simulink model "fixedEEControlR2016a"  (Simulink 8.8)
settings: Solver=ode5  StartTime=0.0  StopTime=inf  FixedStep=0.01  RelTol=1e-3  EnableMultiTasking=on
InitFcn:
  | initFixedEEControl
values from neighbouring files (symbols this model uses):
  WBTConfigRobot = WBToolbox.Configuration    [initEndEffectorControl.m]    (also in initFixedEEControl.m)
undefined symbols (not defined in the file or in its folder): CONFIG, GAINS
libraries: WBToolboxLibrary x19
settings Model: SuppressorTable=22 serialization::archive 11 0 3 0 0 0 11 0  Creator=yeshi  LastModifiedBy=icub  NumberOfSteps=50
settings DataIOCC: LimitDataPoints=off  SaveFormat=Dataset  SignalLoggingSaveFormat=Dataset
settings DebuggingCC: UnderspecifiedInitializationDetection=Simplified  MergeDetectMultiDrivingBlocksExec=error  FcnCallInpInsideContextMsg=error  StateNameClashWarn=none
settings HardwareCC: ProdBitPerPointer=64  ProdBitPerSizeT=64  ProdBitPerPtrDiffT=64  ProdLargestAtomicFloat=Float  ProdIntDivRoundTo=Zero  ProdEndianess=LittleEndian  ProdWordSize=64  ProdHWDeviceType=Intel->x86-64 (Windows64)
settings ModelReferenceCC: PropagateSignalLabelsOutOfModel=on
settings GRTTargetCC: CombineOutputUpdateFcns=on  GRTInterface=off

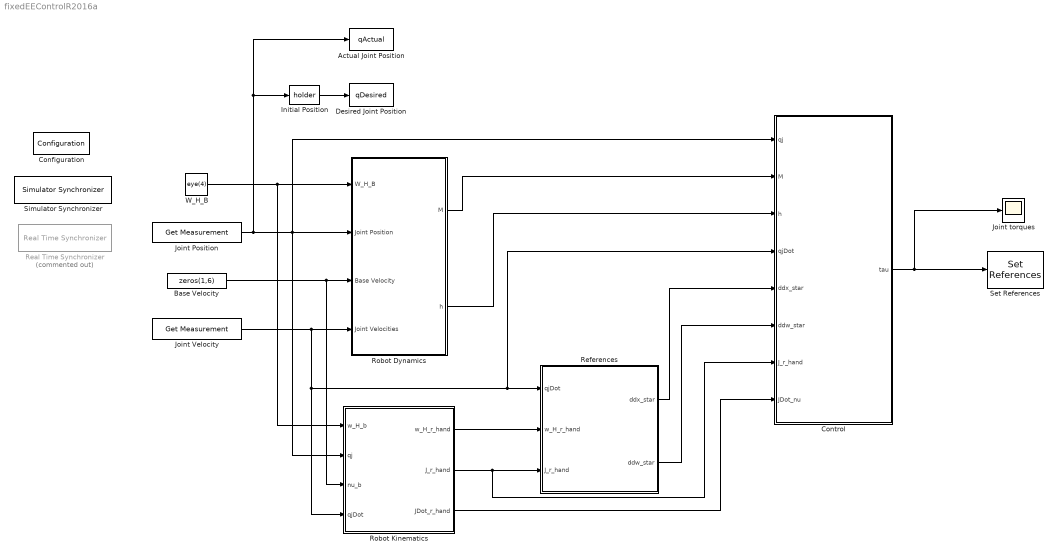
== system fixedEEControlR2016a ==
  Actual Joint Position : ToWorkspace  VariableName=qActual  SaveFormat=Timeseries  SampleTime=-1
  "Base Velocity " : Constant  Value=zeros(1,6)
  Configuration : WBToolboxLibrary/Utilities/Configuration  ConfigSource=Workspace  ConfigObject='WBTConfigRobot'  RobotName='icub'  UrdfFile='model.urdf'  ControlledJoints={'l_elbow','l_shoulder_pitch','torso_roll'}  ControlBoardsNames={'left_arm','right_arm','torso'}  LocalName='WBT'  GravityVector=[0,0,-9.81]
  Control : Subsystem
  Desired Joint Position : ToWorkspace  VariableName=qDesired  SaveFormat=Timeseries  SampleTime=-1
  "Initial Position " : WBToolboxLibrary/Utilities/holder 
  Joint Position : WBToolboxLibrary/wholeBodyStates/Get Measurement  measuredType=Joints Position
  Joint Velocity : WBToolboxLibrary/wholeBodyStates/Get Measurement  measuredType=Joints Velocity
  Joint torques : Scope
  Real Time Synchronizer : WBToolboxLibrary/Utilities/Real Time Synchronizer  Commented=on  period=0.01
  References : Subsystem
  Robot Dynamics : Subsystem
  Robot Kinematics : Subsystem
  Set References : WBToolboxLibrary/wholeBodyActuators/Set References  controlType=Torque  refSpeed=50
  Simulator Synchronizer : WBToolboxLibrary/Utilities/Simulator Synchronizer  period=0.01  serverPortName='/clock/rpc'  clientPortName='/WBT_synchronizer/rpc:o'
  "W_H_B " : Constant  Value=eye(4)
  wires:
  Joint Position/1 -> Robot Kinematics/2(qj), Control/1(qj), Robot Dynamics/2(Joint Position), Actual Joint Position/1, "Initial Position "/1
  Joint Velocity/1 -> Robot Kinematics/4(qjDot), Control/4(qjDot), References/1(qjDot), Robot Dynamics/4(" Joint Velocities ")
  "W_H_B "/1 -> Robot Kinematics/1(w_H_b), Robot Dynamics/1(W_H_B)
  "Base Velocity "/1 -> Robot Kinematics/3(nu_b), Robot Dynamics/3(Base Velocity)
  Robot Kinematics/1(w_H_r_hand) -> References/2(w_H_r_hand)
  Control/1(tau) -> Set References/1, Joint torques/1
  Robot Kinematics/3(JDot_r_hand) -> Control/8(JDot_nu)
  Robot Kinematics/2(J_r_hand) -> References/3(J_r_hand), Control/7(J_r_hand)
  References/1(ddx_star) -> Control/5(ddx_star)
  Robot Dynamics/2(h) -> Control/3(h)
  References/2(ddw_star) -> Control/6(ddw_star)
  "Initial Position "/1 -> Desired Joint Position/1
  Robot Dynamics/1(M) -> Control/2(M)

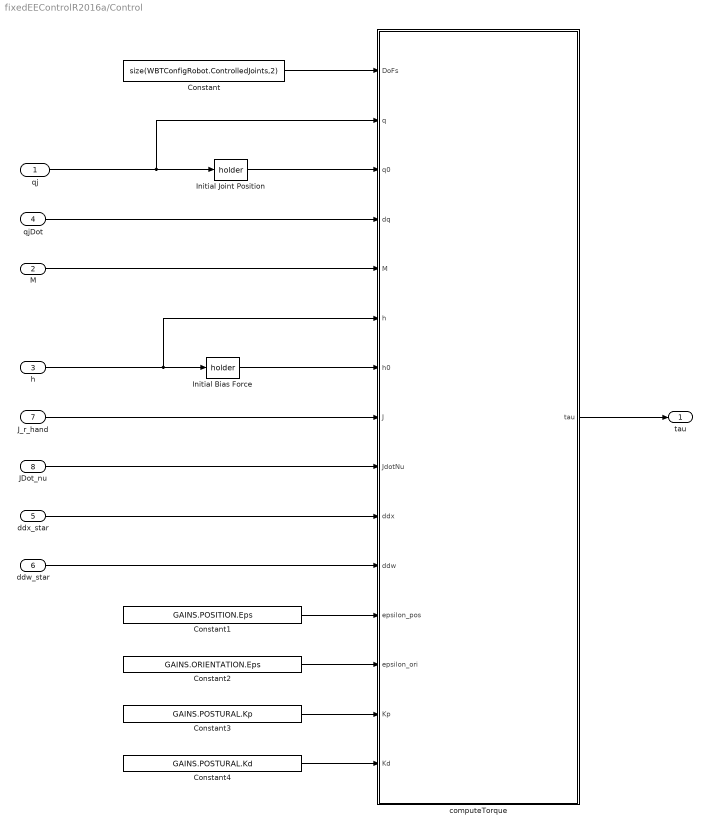
== system fixedEEControlR2016a/Control ==
  qj : Inport
  M : Inport  Port=2
  h : Inport  Port=3
  qjDot : Inport  Port=4
  ddx_star : Inport  Port=5
  ddw_star : Inport  Port=6
  J_r_hand : Inport  Port=7
  JDot_nu : Inport  Port=8
  Constant : Constant  Value=size(WBTConfigRobot.ControlledJoints,2)
  Constant1 : Constant  Value=GAINS.POSITION.Eps
  Constant2 : Constant  Value=GAINS.ORIENTATION.Eps
  Constant3 : Constant  Value=GAINS.POSTURAL.Kp
  Constant4 : Constant  Value=GAINS.POSTURAL.Kd
  Initial Bias Force : WBToolboxLibrary/Utilities/holder 
  Initial Joint Position : WBToolboxLibrary/Utilities/holder 
  computeTorque : MATLAB Function  TreatAsAtomicUnit=on
  tau : Outport
  wires:
  ddx_star/1 -> computeTorque/10(ddx)
  qj/1 -> Initial Joint Position/1, computeTorque/2(q)
  qjDot/1 -> computeTorque/4(dq)
  JDot_nu/1 -> computeTorque/9(JdotNu)
  Constant/1 -> computeTorque/1(DoFs)
  computeTorque/1(tau) -> tau/1
  h/1 -> computeTorque/6(h), Initial Bias Force/1
  Initial Bias Force/1 -> computeTorque/7(h0)
  Initial Joint Position/1 -> computeTorque/3(q0)
  J_r_hand/1 -> computeTorque/8(J)
  M/1 -> computeTorque/5(M)
  ddw_star/1 -> computeTorque/11(ddw)
  Constant1/1 -> computeTorque/12(epsilon_pos)
  Constant2/1 -> computeTorque/13(epsilon_ori)
  Constant3/1 -> computeTorque/14(Kp)
  Constant4/1 -> computeTorque/15(Kd)

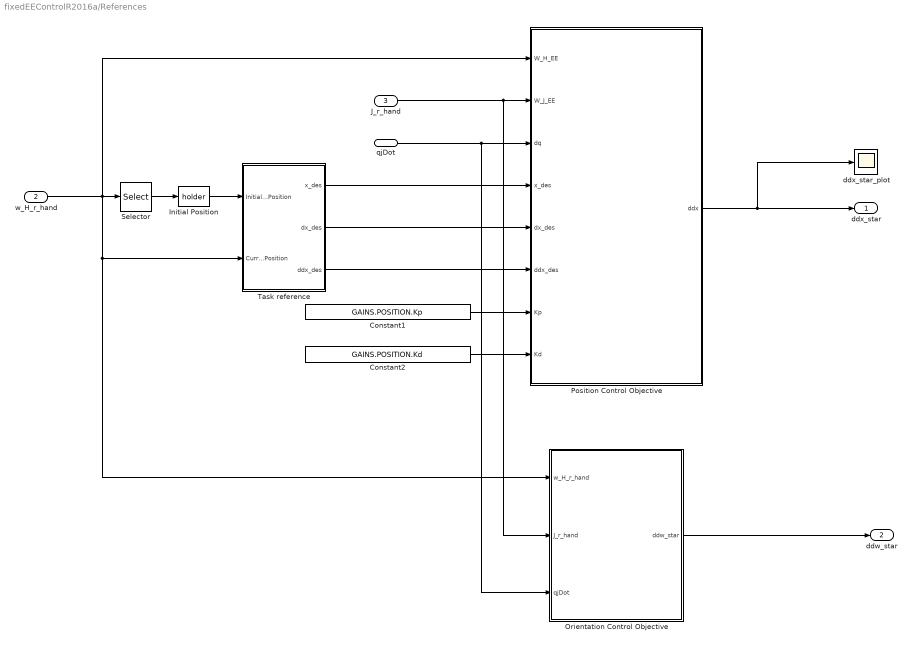
== system fixedEEControlR2016a/References ==
  qjDot : Inport
  w_H_r_hand : Inport  Port=2
  J_r_hand : Inport  Port=3
  Constant1 : Constant  Value=GAINS.POSITION.Kp
  Constant2 : Constant  Value=GAINS.POSITION.Kd
  "Initial Position " : WBToolboxLibrary/Utilities/holder 
  Orientation Control Objective : Subsystem
  Position Control Objective : MATLAB Function  TreatAsAtomicUnit=on
  Selector : Selector  NumberOfDimensions=2  InputPortWidth=3  IndexOptions=Index vector (dialog),Index vector (dialog)  Indices=[1 2 3],4  OutputSizes=1,1
  Task reference : Subsystem
  ddx_star_plot : Scope
  ddx_star : Outport
  ddw_star : Outport  Port=2
  wires:
  J_r_hand/1 -> Orientation Control Objective/2(J_r_hand), Position Control Objective/2(W_J_EE)
  Task reference/1(x_des) -> Position Control Objective/4(x_des)
  Task reference/2(dx_des) -> Position Control Objective/5(dx_des)
  Task reference/3(ddx_des) -> Position Control Objective/6(ddx_des)
  "Initial Position "/1 -> Task reference/1(Initial Position)
  Position Control Objective/1(ddx) -> ddx_star/1, ddx_star_plot/1
  Selector/1 -> "Initial Position "/1
  qjDot/1 -> Orientation Control Objective/3(qjDot), Position Control Objective/3(dq)
  w_H_r_hand/1 -> Selector/1, Position Control Objective/1(W_H_EE), Orientation Control Objective/1(w_H_r_hand), Task reference/2(Current Position)
  Constant1/1 -> Position Control Objective/7(Kp)
  Constant2/1 -> Position Control Objective/8(Kd)
  Orientation Control Objective/1(ddw_star) -> ddw_star/1

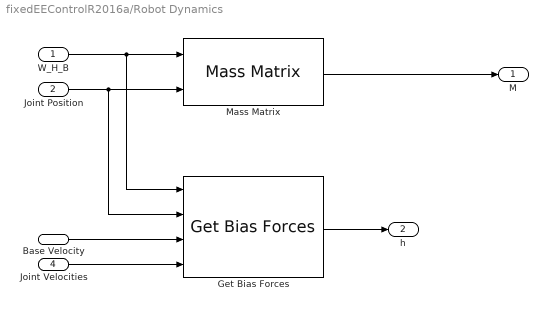
== system fixedEEControlR2016a/Robot Dynamics ==
  W_H_B : Inport
  Joint Position : Inport  Port=2
  Base Velocity : Inport  Port=3
  " Joint Velocities " : Inport  Port=4
  Get Bias Forces : WBToolboxLibrary/wholeBodyModel/Dynamics/Get Bias Forces
  Mass Matrix : WBToolboxLibrary/wholeBodyModel/Dynamics/Mass Matrix
  M : Outport
  h : Outport  Port=2
  wires:
  Joint Position/1 -> Mass Matrix/2, Get Bias Forces/2
  " Joint Velocities "/1 -> Get Bias Forces/4
  Get Bias Forces/1 -> h/1
  W_H_B/1 -> Mass Matrix/1, Get Bias Forces/1
  Base Velocity/1 -> Get Bias Forces/3
  Mass Matrix/1 -> M/1

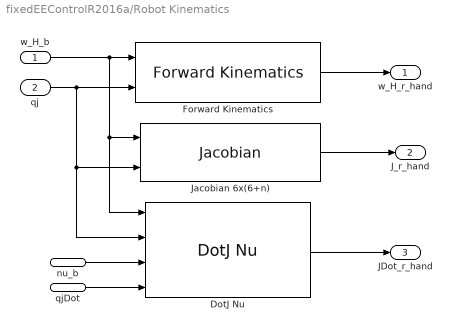
== system fixedEEControlR2016a/Robot Kinematics ==
  w_H_b : Inport
  qj : Inport  Port=2
  nu_b : Inport  Port=3
  qjDot : Inport  Port=4
  DotJ Nu : WBToolboxLibrary/wholeBodyModel/Jacobians/DotJ Nu  frameName=CONFIG.EE
  Forward Kinematics : WBToolboxLibrary/wholeBodyModel/Kinematics/Forward Kinematics  frameName=CONFIG.EE
  Jacobian 6x(6+n) : WBToolboxLibrary/wholeBodyModel/Jacobians/Jacobian  frameName=CONFIG.EE
  w_H_r_hand : Outport
  J_r_hand : Outport  Port=2
  JDot_r_hand : Outport  Port=3
  wires:
  w_H_b/1 -> DotJ Nu/1, Jacobian 6x(6+n)/1, Forward Kinematics/1
  qj/1 -> DotJ Nu/2, Jacobian 6x(6+n)/2, Forward Kinematics/2
  qjDot/1 -> DotJ Nu/4
  nu_b/1 -> DotJ Nu/3
  Jacobian 6x(6+n)/1 -> J_r_hand/1
  Forward Kinematics/1 -> w_H_r_hand/1
  DotJ Nu/1 -> JDot_r_hand/1

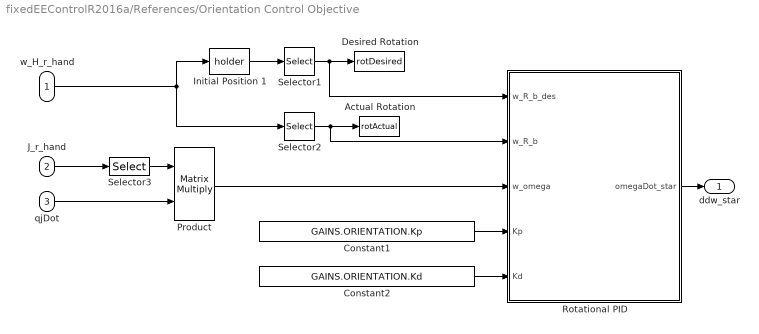
== system fixedEEControlR2016a/References/Orientation Control Objective ==
  w_H_r_hand : Inport
  J_r_hand : Inport  Port=2
  qjDot : Inport  Port=3
  Actual Rotation : ToWorkspace  VariableName=rotActual  SaveFormat=Timeseries  SampleTime=-1
  Constant1 : Constant  Value=GAINS.ORIENTATION.Kp
  Constant2 : Constant  Value=GAINS.ORIENTATION.Kd
  Desired Rotation : ToWorkspace  VariableName=rotDesired  SaveFormat=Timeseries  SampleTime=-1
  Initial Position 1 : WBToolboxLibrary/Utilities/holder 
  Product : Product  Multiplication=Matrix(*)
  Rotational PID : MATLAB Function  TreatAsAtomicUnit=on
  Selector1 : Selector  NumberOfDimensions=2  InputPortWidth=4  IndexOptions=Index vector (dialog),Index vector (dialog)  Indices=[1:3],[1:3]  OutputSizes=1,1
  Selector2 : Selector  NumberOfDimensions=2  InputPortWidth=4  IndexOptions=Index vector (dialog),Index vector (dialog)  Indices=[1:3],[1:3]  OutputSizes=1,1
  Selector3 : Selector  NumberOfDimensions=2  InputPortWidth=4  IndexOptions=Index vector (dialog),Index vector (dialog)  Indices=[4:6],[7:6+13]  OutputSizes=1,1
  ddw_star : Outport
  wires:
  Selector2/1 -> Rotational PID/2(w_R_b), Actual Rotation/1
  Rotational PID/1(omegaDot_star) -> ddw_star/1
  Selector1/1 -> Desired Rotation/1, Rotational PID/1(w_R_b_des)
  w_H_r_hand/1 -> Selector2/1, Initial Position 1/1
  Initial Position 1/1 -> Selector1/1
  Constant1/1 -> Rotational PID/4(Kp)
  Constant2/1 -> Rotational PID/5(Kd)
  J_r_hand/1 -> Selector3/1
  Selector3/1 -> Product/1
  qjDot/1 -> Product/2
  Product/1 -> Rotational PID/3(w_omega)

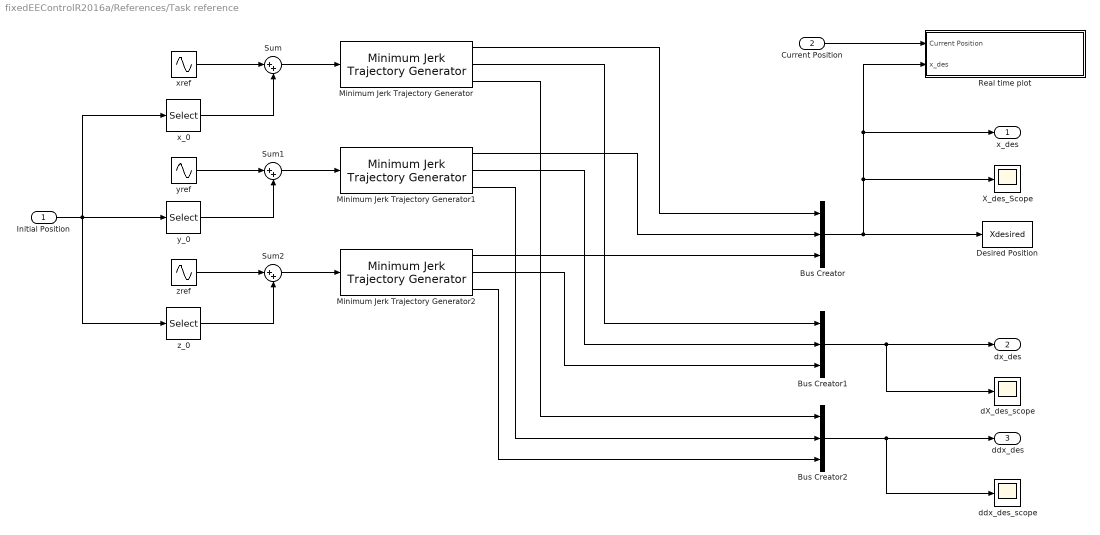
== system fixedEEControlR2016a/References/Task reference ==
  Initial Position : Inport
  Current Position : Inport  Port=2
  Bus Creator : BusCreator  Inputs=3
  Bus Creator1 : BusCreator  Inputs=3
  Bus Creator2 : BusCreator  Inputs=3
  Desired Position : ToWorkspace  VariableName=Xdesired  SaveFormat=Timeseries  SampleTime=-1
  Minimum Jerk Trajectory Generator : WBToolboxLibrary/Utilities/Minimum Jerk Trajectory Generator  externalSettlingTime=off  settlingTime=3  sampleTime=0.01  resetOnSettlingTime=off  firstDerivatives=on  secondDerivatives=on  explicitInitialValue=off
  Minimum Jerk Trajectory Generator1 : WBToolboxLibrary/Utilities/Minimum Jerk Trajectory Generator  externalSettlingTime=off  settlingTime=3  sampleTime=0.01  resetOnSettlingTime=off  firstDerivatives=on  secondDerivatives=on  explicitInitialValue=off
  Minimum Jerk Trajectory Generator2 : WBToolboxLibrary/Utilities/Minimum Jerk Trajectory Generator  externalSettlingTime=off  settlingTime=3  sampleTime=0.01  resetOnSettlingTime=off  firstDerivatives=on  secondDerivatives=on  explicitInitialValue=off
  Real time plot : Subsystem
  Sum : Sum  Inputs=|++
  Sum1 : Sum  Inputs=|++
  Sum2 : Sum  Inputs=|++
  X_des_Scope : Scope
  dX_des_scope : Scope
  ddx_des_scope : Scope
  x_0 : Selector  InputPortWidth=3  IndexOptions=Index vector (dialog)  Indices=[1]  OutputSizes=1
  xref : Sin  Amplitude=0  SampleTime=0
  y_0 : Selector  InputPortWidth=3  IndexOptions=Index vector (dialog)  Indices=[2]  OutputSizes=1
  yref : Sin  Amplitude=0.075  SampleTime=0
  z_0 : Selector  InputPortWidth=3  IndexOptions=Index vector (dialog)  Indices=[3]  OutputSizes=1
  zref : Sin  Amplitude=0.075  Phase=pi/2  SampleTime=0
  x_des : Outport
  dx_des : Outport  Port=2
  ddx_des : Outport  Port=3
  wires:
  Minimum Jerk Trajectory Generator2/2 -> Bus Creator1/3
  Sum2/1 -> Minimum Jerk Trajectory Generator2/1
  Minimum Jerk Trajectory Generator2/1 -> Bus Creator/3
  Minimum Jerk Trajectory Generator/3 -> Bus Creator2/1
  yref/1 -> Sum1/1
  Minimum Jerk Trajectory Generator/1 -> Bus Creator/1
  Minimum Jerk Trajectory Generator1/3 -> Bus Creator2/2
  y_0/1 -> Sum1/2
  Sum1/1 -> Minimum Jerk Trajectory Generator1/1
  Minimum Jerk Trajectory Generator2/3 -> Bus Creator2/3
  Bus Creator1/1 -> dx_des/1, dX_des_scope/1
  zref/1 -> Sum2/1
  Minimum Jerk Trajectory Generator1/2 -> Bus Creator1/2
  Bus Creator2/1 -> ddx_des/1, ddx_des_scope/1
  Bus Creator/1 -> Desired Position/1, Real time plot/2(x_des), x_des/1, X_des_Scope/1
  Minimum Jerk Trajectory Generator1/1 -> Bus Creator/2
  xref/1 -> Sum/1
  Minimum Jerk Trajectory Generator/2 -> Bus Creator1/1
  Sum/1 -> Minimum Jerk Trajectory Generator/1
  z_0/1 -> Sum2/2
  Initial Position/1 -> x_0/1, y_0/1, z_0/1
  x_0/1 -> Sum/2
  Current Position/1 -> Real time plot/1(Current Position)

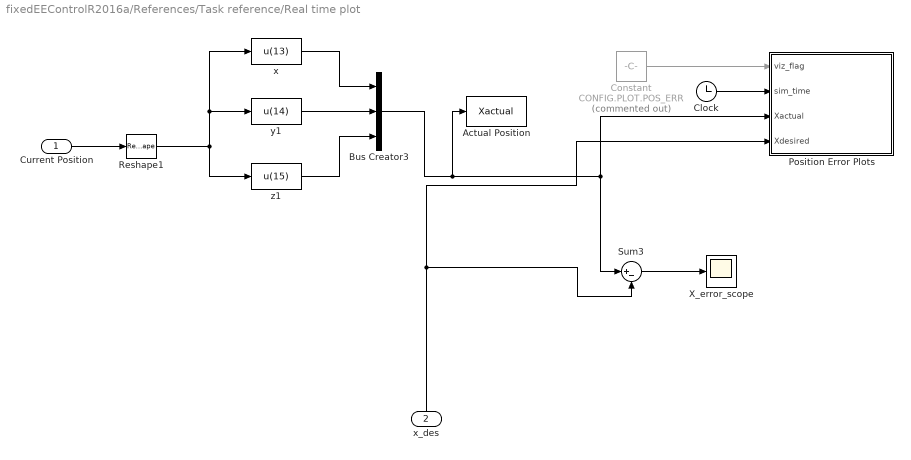
== system fixedEEControlR2016a/References/Task reference/Real time plot ==
  Current Position : Inport
  x_des : Inport  Port=2
  Actual Position : ToWorkspace  VariableName=Xactual  SaveFormat=Timeseries  SampleTime=-1
  Bus Creator3 : BusCreator  Inputs=3
  Clock : Clock
  Constant : Constant  Commented=on  Value=CONFIG.PLOT.POS_ERR
  "Position Error Plots " : MATLAB Function  TreatAsAtomicUnit=on
  Reshape1 : Reshape
  Sum3 : Sum  Inputs=|+-
  X_error_scope : Scope
  x : Fcn  Expr=u(13)
  y1 : Fcn  Expr=u(14)
  z1 : Fcn  Expr=u(15)
  wires:
  x_des/1 -> Sum3/2, "Position Error Plots "/4(Xdesired)
  Current Position/1 -> Reshape1/1
  Reshape1/1 -> x/1, y1/1, z1/1
  x/1 -> Bus Creator3/1
  y1/1 -> Bus Creator3/2
  z1/1 -> Bus Creator3/3
  Clock/1 -> "Position Error Plots "/2(sim_time)
  Bus Creator3/1 -> Actual Position/1, Sum3/1, "Position Error Plots "/3(Xactual)
  Constant/1 -> "Position Error Plots "/1(viz_flag)
  Sum3/1 -> X_error_scope/1

== matlab function References/Position Control Objective ==
  data: W_H_EE input double; ddx output double; W_J_EE input double; dq input double; x_des input double; dx_des input double; ddx_des input double; Kp input double; Kd input double
function ddx = controlObjective(W_H_EE,W_J_EE,dq,x_des,dx_des,ddx_des,Kp,Kd)
   
    x  = W_H_EE(1:3,4)-x_des;
    dx = W_J_EE(1:3,7:end)*dq-dx_des;
    
    ddx = ddx_des-Kp*x-Kd*dx; 

end

== matlab function Control/computeTorque ==
  data: DoFs input double; q input double; q0 input double; dq input double; M input double; h input double; h0 input double; J input double; JdotNu input double; ddx input double; tau output double; ddw input double; epsilon_pos input double; epsilon_ori input double; Kp input double; Kd input double
function tau   = computeTorque(DoFs,q,q0,dq,M,h,h0,J,JdotNu,ddx,ddw,epsilon_pos,epsilon_ori,Kp,Kd)

    Dofs = 13;
    
    Sb = zeros(Dofs,6);
    Ss = eye(Dofs);
    S = [Sb Ss]';

    ddX = [ddx' ddw']';

    %%Position Task
    lambda_pos = (J(1:3,:)/M)*S;
    alpha_pos = pinvDamped(lambda_pos,epsilon_pos);
    
    tau_pos = alpha_pos*(ddX(1:3) - JdotNu(1:3) + (J(1:3,:)/M)*h);
    
    nullspace_pos = eye(size(lambda_pos,2)) - alpha_pos*lambda_pos;
    
    %%Orientation Task
    lambda_ori = (J(4:6,:)/M)*S*nullspace_pos;
    alpha_ori = pinvDamped(lambda_ori,epsilon_ori);
    
    position_bias = (J(4:6,:)/M)*S*tau_pos;
    tau_ori = alpha_ori*(ddX(4:6) - JdotNu(4:6) + (J(4:6,:)/M)*h - position_bias);
    
    nullspace_ori = eye(size(lambda_ori,2)) - alpha_ori*lambda_ori;
    
    %%Second Approach
    kp = Kp;
    kd = Kd;
    tau_null = S'*h - kp*(q-q0) - kd*(dq);
    
% %     tau = tau_pos + nullspace_pos*tau_null;
    tau = tau_pos + nullspace_pos*(tau_ori + nullspace_ori*tau_null);

end

== matlab function References/Task reference/Real time plot/Position Error Plots  ==
  data: viz_flag input double; sim_time input double; Xactual input double; Xdesired input double
function positionErrorPlots(viz_flag,sim_time,Xactual,Xdesired)
%#codegen

coder.extrinsic('animatedline')
coder.extrinsic('addpoints')
coder.extrinsic('legend')
coder.extrinsic('clearpoints')

if(viz_flag ~= 0)
    
    Xerror = Xactual - Xdesired;
    curve_position_error = animatedline('LineWidth',0.1,'Marker','+');

    if(sim_time == 0)
    
        clf;
        close;
    
        fig1 = figure;
        view(177,15); hold on;
        grid on;
        xlabel('x');
        ylabel('y');
        zlabel('z');
        title('Position Error'); hold on;
% %         axis([-0.3 0.3 -0.3 0.3 -0.3 0.3]);
       
    end
    
    figure(1);
    addpoints(curve_position_error,Xerror(1),Xerror(2),Xerror(3));
    drawnow;
    
end

end

== matlab function References/Orientation Control Objective/Rotational PID ==
  data: w_R_b_des input double; w_R_b input double; w_omega input double; omegaDot_star output double; Kp input double; Kd input double
function omegaDot_star = rotPID(w_R_b_des,w_R_b,w_omega,Kp,Kd)

    w_omega_des = [0;0;0];
    w_omegaDot_des = [0;0;0];
    
    omegaDot_star = rotationalPID(w_R_b,w_omega,w_R_b_des,w_omega_des,w_omegaDot_des,Kp,Kd);
end
